simulink model "Fridge_Faulty_27"  (R2024a)
settings: Solver=VariableStepAuto  StartTime=0.0  StopTime=30  RelTol=1e-3
undefined symbols (not defined in the file): sigbuilder_block
settings Model: Creator=aarrieta  LastModifiedBy=airshad
settings SolverCC: AlgebraicLoopSolver=TrustRegion
settings OptimizationCC: ReuseModelBlockBuffer=off
settings DebuggingCC: UnconnectedInputMsg=warning  UnconnectedOutputMsg=warning  UnconnectedLineMsg=warning
settings ModelReferenceCC: EnableRefExpFcnMdlSchedulingChecks=on
settings RTWCC: GPUComputeCapability=3.5  DLArmComputeVersion=19.05

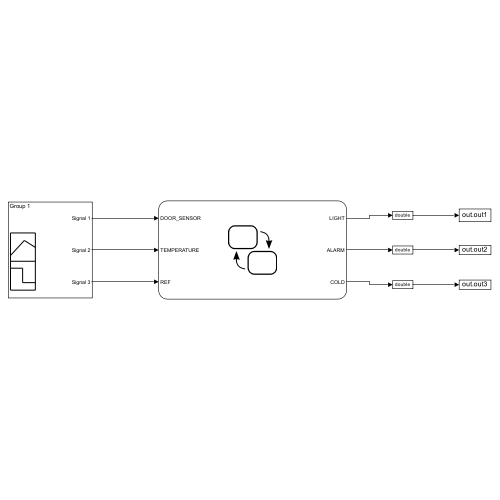
[thumbnail: Simulink's stored preview of the top-level diagram]
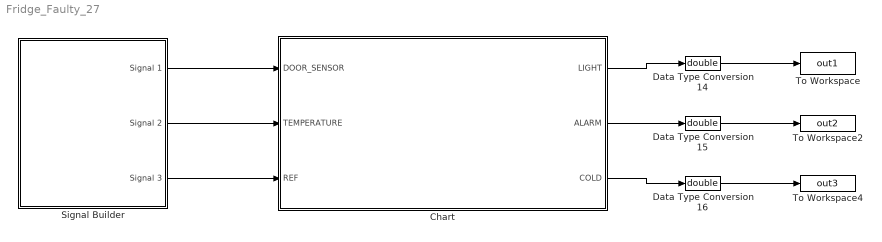
== system Fridge_Faulty_27 ==
  Chart : Stateflow chart  TreatAsAtomicUnit=on
  Data Type Conversion14 : DataTypeConversion  OutDataTypeStr=double  SaturateOnIntegerOverflow=off  RndMeth=Floor
  Data Type Conversion15 : DataTypeConversion  OutDataTypeStr=double  SaturateOnIntegerOverflow=off  RndMeth=Floor
  Data Type Conversion16 : DataTypeConversion  OutDataTypeStr=double  SaturateOnIntegerOverflow=off  RndMeth=Floor
  Signal Builder : Subsystem  Tag=STV Subsys  LoadFcn=sigbuilder_block('load');  StartFcn=sigbuilder_block('start');  StopFcn=sigbuilder_block('stop');  ClipboardFcn=sigbuilder_block('clipboard');  mask(Sigbuilder block){tuvar=[0:10]}
      mask help: Simulink:masks:SigbuilderBlock_MD
      mask init:
      | if ~strcmp(get_param(bdroot(gcbh),'SimulationStatus'),'stopped') tuvar = sigbuilder_block('maskInit'); end
      settings: CopyFcn=sigbuilder_block('copy');  DeleteFcn=sigbuilder_block('delete');  ModelCloseFcn=sigbuilder_block('modelClose');  PreSaveFcn=sigbuilder_block('preSave');  PauseFcn=sigbuilder_block('pause');  ContinueFcn=sigbuilder_block('continue');  NameChangeFcn=sigbuilder_block('namechange');  OpenFcn=sigbuilder_block('open',[438.6 40.8 550.8 400.2 ]);  CloseFcn=sigbuilder_block('close');
      mask Display: plot(0, 0, 100, 100,[2, 2, 32, 32, 2], [68, 8, 8, 68, 68],[32, 2], [38, 38], [32, 19, 2],[53, 60, 44], [32, 17, 17, 2],[16, 16, 31, 31]);txt = getActiveGroup(gcbh);text(2, 100, txt,'verticalAlignment', 'top');
  To Workspace : ToWorkspace  VariableName=out1  SaveFormat=Timeseries  SampleTime=-1
  To Workspace2 : ToWorkspace  VariableName=out2  SaveFormat=Timeseries  SampleTime=-1
  To Workspace4 : ToWorkspace  VariableName=out3  SaveFormat=Timeseries  SampleTime=-1
  wires:
  Chart/3(COLD) -> Data Type Conversion16/1
  Data Type Conversion16/1 -> To Workspace4/1
  Data Type Conversion15/1 -> To Workspace2/1
  Chart/2(ALARM) -> Data Type Conversion15/1
  Chart/1(LIGHT) -> Data Type Conversion14/1
  Data Type Conversion14/1 -> To Workspace/1
  Signal Builder/2(Signal 2) -> Chart/2(TEMPERATURE)
  Signal Builder/1(Signal 1) -> Chart/1(DOOR_SENSOR)
  Signal Builder/3(Signal 3) -> Chart/3(REF)

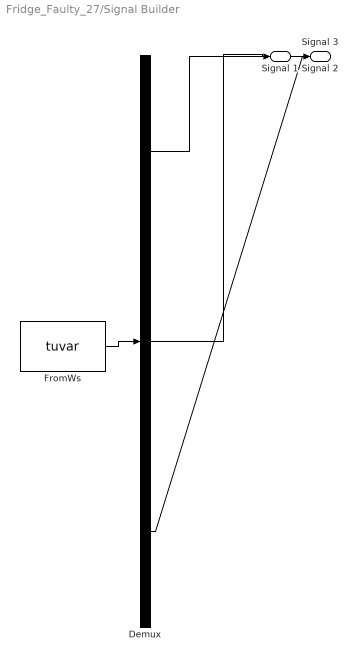
== system Fridge_Faulty_27/Signal Builder ==
  Demux : Demux  Tag=STV Demux  Outputs=3
      settings: DisplayOption=none
  FromWs : FromWorkspace  Tag=STV FromWs  VariableName=tuvar
      SigBuilderData=|
      | common.afterFinalStr = 'Extrapolate'
      | common.sampleTime = 0
      | dataSet(1).timeRange = [0 30]
      | dataSet(1).name = 'Group 1'
      | dataSet(2).timeRange = [0 30]
      | dataSet(2).name = 'Group 2'
      | sbobj.Groups(1).Name = 'Group 1'
      | sbobj.Groups(1).Signals(1).Name = 'Signal 1'
      | sbobj.Groups(1).Signals(1).XData = [0 4 6 30]
      | sbobj.Groups(1).Signals(1).YData = [0 0 0 0]
      | sbobj.Groups(1).Signals(2).Name = 'Signal 2'
      | sbobj.Groups(1).Signals(2).XData = [0 4 4 10.3 10.3 30]
      | sbobj.Groups(1).Signals(2).YData = [0 0 10 10 0 0]
      | sbobj.Groups(1).Signals(3).Name = 'Signal 3'
      | sbobj.Groups(1).Signals(3).XData = [0 4 4 10.2 10.2 30]
      | sbobj.Groups(1).Signals(3).YData = [0 0 1 1 0 0]
      | sbobj.Groups(1).TimeRange = [0 30]
      | sbobj.Groups(2).Name = 'Group 2'
      | sbobj.Groups(2).Signals(1).Name = 'Signal 1'
      | sbobj.Groups(2).Signals(1).XData = [0 4 6 30]
      | sbobj.Groups(2).Signals(1).YData = [1 1 1 1]
      | sbobj.Groups(2).Signals(2).Name = 'Signal 2'
      | sbobj.Groups(2).Signals(2).XData = [0 4 4 10.3 10.3 30]
      | sbobj.Groups(2).Signals(2).YData = [0 0 10 10 0 0]
      | sbobj.Groups(2).Signals(3).Name = 'Signal 3'
      | sbobj.Groups(2).Signals(3).XData = [0 4 4 10.2 10.2 30]
      | sbobj.Groups(2).Signals(3).YData = [0 0 1 1 0 0]
      | sbobj.Groups(2).TimeRange = [0 30]
  Signal 1 : Outport  Tag=STV Outport
  Signal 2 : Outport  Tag=STV Outport  Port=2
  Signal 3 : Outport  Tag=STV Outport  Port=3
  wires:
  Demux/1 -> Signal 1/1
  FromWs/1 -> Demux/1
  Demux/2 -> Signal 2/1
  Demux/3 -> Signal 3/1

== stateflow chart Fridge_Faulty_27/Chart ==
  state OPEN
    during:
    LIGHT = 1;
    ALARM =0;
    COLD = 0;
  state CLOSE_NORM
    during:
    LIGHT = 0;
    ALARM = 0;
    COLD = 0;
  state OPEN_15_SEC
    during:
    LIGHT = 1;
    ALARM = 1;
  state CLOSE_HOTduring_COLD = REF - TEMPERATURE;
  OPEN_15_SEC -> CLOSE_NORM : [DOOR_SENSOR == 0]
  (default) -> CLOSE_NORM
  CLOSE_NORM -> OPEN [order 1] : [DOOR_SENSOR ==1]
  OPEN -> OPEN_15_SEC [order 1] : [after(15,sec)]
  OPEN -> CLOSE_NORM [order 2] : [DOOR_SENSOR == 0]
  CLOSE_HOTduring_COLD = REF - TEMPERATURE; -> OPEN [order 2] : [DOOR_SENSOR ==1]
  CLOSE_HOTduring_COLD = REF - TEMPERATURE; -> CLOSE_NORM [order 1] : [TEMPERATURE <= REF]
  CLOSE_NORM -> CLOSE_HOTduring_COLD = REF - TEMPERATURE; [order 2] : [TEMPERATURE > REF + 2]
  data: LIGHT output; ALARM output; COLD output; DOOR_SENSOR input; TEMPERATURE input; REF input
